simulink library "INT_CoVeh_CalcTrqPrpLimErr"  (R2016b)
settings: Solver=VariableStepAuto  StartTime=0.0  StopTime=10.0  RelTol=1e-3
settings Model: Creator=zhoutinglin  LastModifiedBy=zhoutinglin

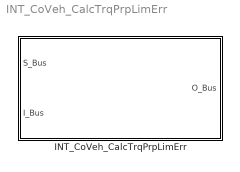
== system INT_CoVeh_CalcTrqPrpLimErr ==
  INT_CoVeh_CalcTrqPrpLimErr : Subsystem

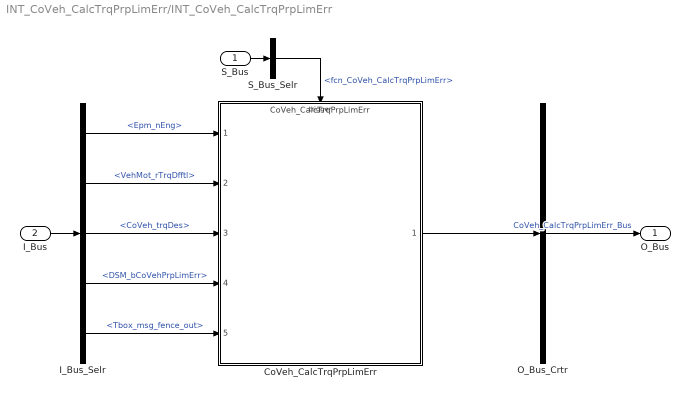
== system INT_CoVeh_CalcTrqPrpLimErr/INT_CoVeh_CalcTrqPrpLimErr ==
  S_Bus : Inport
  I_Bus : Inport  Port=2
  CoVeh_CalcTrqPrpLimErr : ModelReference  ModelNameDialog=CoVeh_CalcTrqPrpLimErr  SimulationMode=Normal  ModelReferenceVersion=1.27  TriggerPortName=function  TriggerPortTriggerType=function-call  TriggerPortStatesWhenEnabling=held
  I_Bus_Selr : BusSelector  OutputSignals=Epm_nEng,VehMot_rTrqDfftl,CoVeh_trqDes,DSM_bCoVehPrpLimErr,Tbox_msg_fence_out
  O_Bus_Crtr : BusCreator  Inputs=1
  S_Bus_Selr : BusSelector  OutputSignals=fcn_CoVeh_CalcTrqPrpLimErr
  O_Bus : Outport
  wires:
  S_Bus_Selr/1 -> CoVeh_CalcTrqPrpLimErr/Trigger  "<fcn_CoVeh_CalcTrqPrpLimErr>"
  S_Bus/1 -> S_Bus_Selr/1
  I_Bus/1 -> I_Bus_Selr/1
  I_Bus_Selr/1 -> CoVeh_CalcTrqPrpLimErr/1  "<Epm_nEng>"
  I_Bus_Selr/2 -> CoVeh_CalcTrqPrpLimErr/2  "<VehMot_rTrqDfftl>"
  I_Bus_Selr/3 -> CoVeh_CalcTrqPrpLimErr/3  "<CoVeh_trqDes>"
  I_Bus_Selr/4 -> CoVeh_CalcTrqPrpLimErr/4  "<DSM_bCoVehPrpLimErr>"
  I_Bus_Selr/5 -> CoVeh_CalcTrqPrpLimErr/5  "<Tbox_msg_fence_out>"
  O_Bus_Crtr/1 -> O_Bus/1  "CoVeh_CalcTrqPrpLimErr_Bus"
  CoVeh_CalcTrqPrpLimErr/1 -> O_Bus_Crtr/1
